simulink library "halin"  (R2021b)
settings: Solver=VariableStepAuto  StartTime=0.0  StopTime=10.0  RelTol=1e-3
undefined symbols (not defined in the file): KHAL_CAN1ABM1E2E_flg, KHAL_CAN1ESC1E2E_flg, KHAL_CAN1ESC5E2E_flg, KHAL_CAN1ESC7E2E_flg, KHAL_CAN1FCM2E2E_flg, KHAL_CAN1FCM3E2E_flg, KHAL_CAN1FCM4E2E_flg, KHAL_CAN3BMS1E2E_flg, KHAL_CAN3BMS6E2E_flg, KHAL_CAN3CCU1E2E_flg, KHAL_CAN3CCU2E2E_flg, KHAL_CAN3MCUF1E2E_flg, KHAL_CAN3MCUR1E2E_flg, KHAL_CAN3Shifter1E2E_flg, TRUE
libraries: simulink x420, FVT_lib x149, hcu_lib x49
(part 10 of 14)

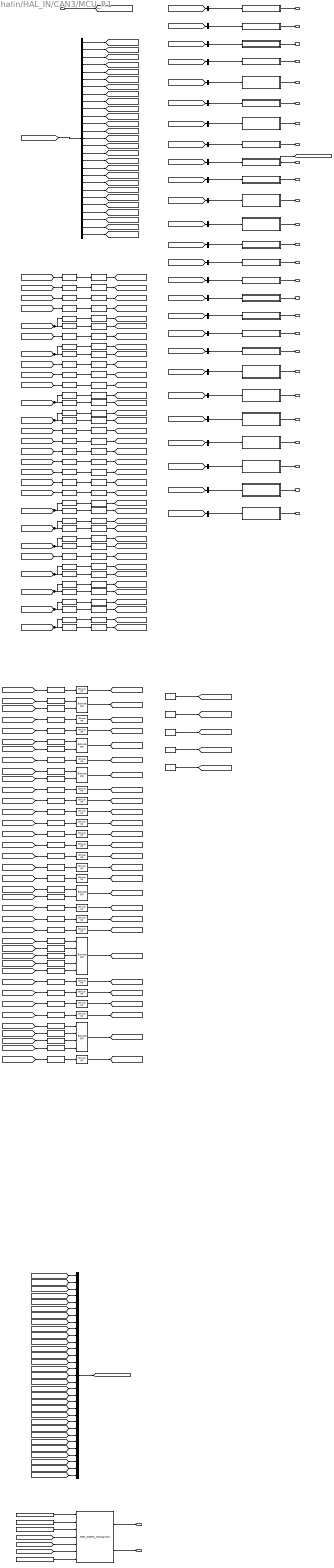
== system halin/HAL_IN/CAN3/MCU_R1 ==
  DT_CAN3_SG_MCU_R1 : Inport
  0x02 : Constant  Value=0x02
  0x78 : Constant  Value=0x78
  BitwiseAND{,1..37} (38 alike) : simulink/Logic and Bit Operations/Bitwise Operator  logicop=AND  UseBitMask=on  BitMask=0xFF  BitMaskRealWorld=Stored Integer
  BitwiseOR{,2..3,5,7..15,17..19,21..24,26} (21 alike) : simulink/Logic and Bit Operations/Bitwise Operator  logicop=OR  UseBitMask=off  BitMask=bin2dec('11011001')  BitMaskRealWorld=Stored Integer
  BitwiseOR{1,4,6,16} (4 alike) : simulink/Logic and Bit Operations/Bitwise Operator  logicop=OR  UseBitMask=off  NumInputPorts=2  BitMask=bin2dec('11011001')  BitMaskRealWorld=Stored Integer
  BitwiseOR20 : simulink/Logic and Bit Operations/Bitwise Operator  logicop=OR  UseBitMask=off  NumInputPorts=5  BitMask=bin2dec('11011001')  BitMaskRealWorld=Stored Integer
  BitwiseOR25 : simulink/Logic and Bit Operations/Bitwise Operator  logicop=OR  UseBitMask=off  NumInputPorts=4  BitMask=bin2dec('11011001')  BitMaskRealWorld=Stored Integer
  DDM_CS&RC_Comparison : FVT_lib/hal/DDM_CS&RC_Comparison  MsgCycleTime=10
  Data Type Conversion{,1..37} (38 alike) : DataTypeConversion  OutDataTypeStr=uint8
  KHAL_CAN3MCUR1E2E_flg : Constant  Value=KHAL_CAN3MCUR1E2E_flg
  LeftShift{,5,7,10..11,13..14} (7 alike) : ArithShift  BitShiftDirection=Left
  LeftShift1 : ArithShift  BitShiftNumber=1  BitShiftDirection=Left
  LeftShift12 : ArithShift  BitShiftNumber=7  BitShiftDirection=Left
  LeftShift15 : ArithShift  BitShiftNumber=1  BitShiftDirection=Left
  LeftShift2 : ArithShift  BitShiftNumber=2  BitShiftDirection=Left
  LeftShift3 : ArithShift  BitShiftNumber=5  BitShiftDirection=Left
  LeftShift4 : ArithShift  BitShiftNumber=6  BitShiftDirection=Left
  LeftShift6 : ArithShift  BitShiftNumber=4  BitShiftDirection=Left
  LeftShift8 : ArithShift  BitShiftNumber=3  BitShiftDirection=Left
  LeftShift9 : ArithShift  BitShiftNumber=4  BitShiftDirection=Left
  MCUWarnR : Subsystem
  MessageRollingCounter : FVT_lib/hal/MessageRollingCounter  CounterMAX=14  task_time_ms=5  msg_time_ms=10
  Mux : Mux  Inputs=31
  RightShift{,2,4,6,10,14,16,18,20} (9 alike) : ArithShift  BitShiftNumber=8
  RightShift{1,3,5,7,11,15,17,19,21} (9 alike) : ArithShift
  RightShift12 : ArithShift  BitShiftNumber=4
  RightShift13 : ArithShift  BitShiftNumber=-4
  RightShift8 : ArithShift  BitShiftNumber=1
  RightShift9 : ArithShift  BitShiftNumber=-7
  RrActvDmpDisabSta : Subsystem
  RrEDUDrtSta : Subsystem
  RrEDUOpratingSta : Subsystem
  RrEDURealTMTq : Subsystem
  RrEDURotateDirction : Subsystem
  RrEDUTqReqFbk : Subsystem
  RrMCU1Chksum : Subsystem
  RrMCU1RolCnt : Subsystem
  RrMCUBAT : Subsystem
  RrMCUDCBusCurr : Subsystem
  RrMCUDCBusVolt : Subsystem
  RrMCUDischrgSta : Subsystem
  RrMCUEnaSta : Subsystem
  RrMCUErr : Subsystem
  RrMCUIGNsta : Subsystem
  RrMCUReady : Subsystem
  RrMCUReady4Pre : Subsystem
  RrMCUSysSta : Subsystem
  RrMCUTemp : Subsystem
  RrMotorAvailTq : Subsystem
  RrRegenAvailTq : Subsystem
  RrTMSpd : Subsystem
  RrTMTemp : Subsystem
  RrTMid : Subsystem
  RrTMiq : Subsystem
  bus_selector : BusSelector  OutputSignals=CAN3_MCUWarn_R,CAN3_Rr_ActvDmpDisabSta,CAN3_Rr_EDUDrtSta,CAN3_Rr_EDUOpratingSta,CAN3_Rr_EDURealTMTq,CAN3_Rr_EDURotateDirction,CAN3_Rr_EDUTqReqFbk,CAN3_Rr_MCU1Chksum,CAN3_Rr_MCU1RolCnt,CAN3_Rr_MCUBAT,CAN3_Rr_MCUDCBusCurr,CAN3_Rr_MCUDCBusVolt,CAN3_Rr_MCUDischrgSta,CAN3_Rr_MCUEnaSta,CAN3_Rr_MCUErr,CAN3_Rr_MCUIGN_sta,CAN3_Rr_MCUReady,CAN3_Rr_MCUReady4Pre,CAN3_Rr_MCUSysSta,CAN3_Rr_MCUTemp,CAN3_Rr_MotorAvailTq,CAN3_Rr_RegenAvailTq,CAN3_Rr_Reserved_bits,CAN3_Rr_TMSpd,CAN3_Rr_TMTemp,CAN3_Rr_TMid,CAN3_Rr_TMiq
  bus_selector1 : BusSelector  OutputSignals=CAN3_MCUWarn_R
  bus_selector10 : BusSelector  OutputSignals=CAN3_Rr_MCUBAT
  bus_selector11 : BusSelector  OutputSignals=CAN3_Rr_MCUDCBusCurr
  bus_selector12 : BusSelector  OutputSignals=CAN3_Rr_MCUDCBusVolt
  bus_selector13 : BusSelector  OutputSignals=CAN3_Rr_MCUDischrgSta
  bus_selector14 : BusSelector  OutputSignals=CAN3_Rr_MCUEnaSta
  bus_selector15 : BusSelector  OutputSignals=CAN3_Rr_MCUErr
  bus_selector16 : BusSelector  OutputSignals=CAN3_Rr_MCUIGN_sta
  bus_selector17 : BusSelector  OutputSignals=CAN3_Rr_MCUReady
  bus_selector18 : BusSelector  OutputSignals=CAN3_Rr_MCUReady4Pre
  bus_selector19 : BusSelector  OutputSignals=CAN3_Rr_MCUSysSta
  bus_selector2 : BusSelector  OutputSignals=CAN3_Rr_ActvDmpDisabSta
  bus_selector20 : BusSelector  OutputSignals=CAN3_Rr_MCUTemp
  bus_selector21 : BusSelector  OutputSignals=CAN3_Rr_MotorAvailTq
  bus_selector22 : BusSelector  OutputSignals=CAN3_Rr_RegenAvailTq
  bus_selector23 : BusSelector  OutputSignals=CAN3_Rr_TMSpd
  bus_selector24 : BusSelector  OutputSignals=CAN3_Rr_TMTemp
  bus_selector25 : BusSelector  OutputSignals=CAN3_Rr_TMid
  bus_selector26 : BusSelector  OutputSignals=CAN3_Rr_TMiq
  bus_selector3 : BusSelector  OutputSignals=CAN3_Rr_EDUDrtSta
  bus_selector4 : BusSelector  OutputSignals=CAN3_Rr_EDUOpratingSta
  bus_selector5 : BusSelector  OutputSignals=CAN3_Rr_EDURealTMTq
  bus_selector6 : BusSelector  OutputSignals=CAN3_Rr_EDURotateDirction
  bus_selector7 : BusSelector  OutputSignals=CAN3_Rr_EDUTqReqFbk
  bus_selector8 : BusSelector  OutputSignals=CAN3_Rr_MCU1Chksum
  bus_selector9 : BusSelector  OutputSignals=CAN3_Rr_MCU1RolCnt
  constant{,1..4} (5 alike) : Constant  Value=0x0  OutDataTypeStr=uint8
  VHAL_MCUR1CSErr_flg : Outport
  VHAL_MCUR1RCErr_flg : Outport  Port=2
  VHAL_MCUWarnR_enum : Outport  Port=3
  VHAL_RrActvDmpDisabSta_flg : Outport  Port=4
  VHAL_RrEDUDrtSta_flg : Outport  Port=5
  VHAL_RrEDUOpratingSta_flg : Outport  Port=6
  VHAL_RrEDURealTMTq_Nm : Outport  Port=7
  VHAL_RrEDURotateDirction_enum : Outport  Port=8
  VHAL_RrEDUTqReqFbk_Nm : Outport  Port=9
  VHAL_RrMCU1Chksum_enum : Outport  Port=10
  VHAL_RrMCU1RolCnt_enum : Outport  Port=11
  VHAL_RrMCUBAT_V : Outport  Port=12
  VHAL_RrMCUDCBusCurr_A : Outport  Port=13
  VHAL_RrMCUDCBusVolt_V : Outport  Port=14
  VHAL_RrMCUDischrgSta_flg : Outport  Port=15
  VHAL_RrMCUEnaSta_flg : Outport  Port=16
  VHAL_RrMCUErr_enum : Outport  Port=17
  VHAL_RrMCUIGNsta_flg : Outport  Port=18
  VHAL_RrMCUReady_flg : Outport  Port=19
  VHAL_RrMCUReady4Pre_flg : Outport  Port=20
  VHAL_RrMCUSysSta_enum : Outport  Port=21
  VHAL_RrMCUTemp_C : Outport  Port=22
  VHAL_RrMotorAvailTq_Nm : Outport  Port=23
  VHAL_RrRegenAvailTq_Nm : Outport  Port=24
  VHAL_RrTMSpd_rpm : Outport  Port=25
  VHAL_RrTMTemp_C : Outport  Port=26
  VHAL_RrTMid_A : Outport  Port=27
  VHAL_RrTMiq_A : Outport  Port=28
  wires:
  DT_CAN3_SG_MCU_R1/1 -> [DT_CAN3_SG_MCU_R1]
  [DT_CAN3_SG_MCU_R1] -> bus_selector/1
  bus_selector/1 -> [CAN3_MCUWarn_R]  "<CAN3_MCUWarn_R>"
  [CAN3_MCUWarn_R] -> LeftShift/1
  LeftShift/1 -> BitwiseAND/1
  BitwiseAND/1 -> [Byte_1_CAN3_MCUWarn_R]
  bus_selector/2 -> [CAN3_Rr_ActvDmpDisabSta]  "<CAN3_Rr_ActvDmpDisabSta>"
  [CAN3_Rr_ActvDmpDisabSta] -> LeftShift1/1
  LeftShift1/1 -> BitwiseAND1/1
  BitwiseAND1/1 -> [Byte_25_CAN3_Rr_ActvDmpDisabSta]
  bus_selector/3 -> [CAN3_Rr_EDUDrtSta]  "<CAN3_Rr_EDUDrtSta>"
  [CAN3_Rr_EDUDrtSta] -> LeftShift2/1
  LeftShift2/1 -> BitwiseAND2/1
  BitwiseAND2/1 -> [Byte_25_CAN3_Rr_EDUDrtSta]
  bus_selector/4 -> [CAN3_Rr_EDUOpratingSta]  "<CAN3_Rr_EDUOpratingSta>"
  [CAN3_Rr_EDUOpratingSta] -> LeftShift3/1
  LeftShift3/1 -> BitwiseAND3/1
  BitwiseAND3/1 -> [Byte_30_CAN3_Rr_EDUOpratingSta]
  bus_selector/5 -> [CAN3_Rr_EDURealTMTq]  "<CAN3_Rr_EDURealTMTq>"
  [CAN3_Rr_EDURealTMTq] -> RightShift/1, RightShift1/1
  RightShift/1 -> BitwiseAND4/1
  BitwiseAND4/1 -> [Byte_28_CAN3_Rr_EDURealTMTq]
  RightShift1/1 -> BitwiseAND5/1
  BitwiseAND5/1 -> [Byte_29_CAN3_Rr_EDURealTMTq]
  bus_selector/6 -> [CAN3_Rr_EDURotateDirction]  "<CAN3_Rr_EDURotateDirction>"
  [CAN3_Rr_EDURotateDirction] -> LeftShift4/1
  LeftShift4/1 -> BitwiseAND6/1
  BitwiseAND6/1 -> [Byte_30_CAN3_Rr_EDURotateDirction]
  bus_selector/7 -> [CAN3_Rr_EDUTqReqFbk]  "<CAN3_Rr_EDUTqReqFbk>"
  [CAN3_Rr_EDUTqReqFbk] -> RightShift2/1, RightShift3/1
  RightShift2/1 -> BitwiseAND7/1
  BitwiseAND7/1 -> [Byte_30_CAN3_Rr_EDUTqReqFbk]
  RightShift3/1 -> BitwiseAND8/1
  BitwiseAND8/1 -> [Byte_31_CAN3_Rr_EDUTqReqFbk]
  bus_selector/8 -> [CAN3_Rr_MCU1Chksum]  "<CAN3_Rr_MCU1Chksum>"
  [CAN3_Rr_MCU1Chksum] -> LeftShift5/1
  LeftShift5/1 -> BitwiseAND9/1
  BitwiseAND9/1 -> [Byte_0_CAN3_Rr_MCU1Chksum]
  bus_selector/9 -> [CAN3_Rr_MCU1RolCnt]  "<CAN3_Rr_MCU1RolCnt>"
  [CAN3_Rr_MCU1RolCnt] -> LeftShift6/1
  LeftShift6/1 -> BitwiseAND10/1
  BitwiseAND10/1 -> [Byte_1_CAN3_Rr_MCU1RolCnt]
  bus_selector/10 -> [CAN3_Rr_MCUBAT]  "<CAN3_Rr_MCUBAT>"
  [CAN3_Rr_MCUBAT] -> LeftShift7/1
  LeftShift7/1 -> BitwiseAND11/1
  BitwiseAND11/1 -> [Byte_8_CAN3_Rr_MCUBAT]
  bus_selector/11 -> [CAN3_Rr_MCUDCBusCurr]  "<CAN3_Rr_MCUDCBusCurr>"
  [CAN3_Rr_MCUDCBusCurr] -> RightShift4/1, RightShift5/1
  RightShift4/1 -> BitwiseAND12/1
  BitwiseAND12/1 -> [Byte_21_CAN3_Rr_MCUDCBusCurr]
  RightShift5/1 -> BitwiseAND13/1
  BitwiseAND13/1 -> [Byte_22_CAN3_Rr_MCUDCBusCurr]
  bus_selector/12 -> [CAN3_Rr_MCUDCBusVolt]  "<CAN3_Rr_MCUDCBusVolt>"
  [CAN3_Rr_MCUDCBusVolt] -> RightShift6/1, RightShift7/1
  RightShift6/1 -> BitwiseAND14/1
  BitwiseAND14/1 -> [Byte_23_CAN3_Rr_MCUDCBusVolt]
  RightShift7/1 -> BitwiseAND15/1
  BitwiseAND15/1 -> [Byte_24_CAN3_Rr_MCUDCBusVolt]
  bus_selector/13 -> [CAN3_Rr_MCUDischrgSta]  "<CAN3_Rr_MCUDischrgSta>"
  [CAN3_Rr_MCUDischrgSta] -> LeftShift8/1
  LeftShift8/1 -> BitwiseAND16/1
  BitwiseAND16/1 -> [Byte_25_CAN3_Rr_MCUDischrgSta]
  bus_selector/14 -> [CAN3_Rr_MCUEnaSta]  "<CAN3_Rr_MCUEnaSta>"
  [CAN3_Rr_MCUEnaSta] -> LeftShift9/1
  LeftShift9/1 -> BitwiseAND17/1
  BitwiseAND17/1 -> [Byte_30_CAN3_Rr_MCUEnaSta]
  bus_selector/15 -> [CAN3_Rr_MCUErr]  "<CAN3_Rr_MCUErr>"
  [CAN3_Rr_MCUErr] -> LeftShift10/1
  LeftShift10/1 -> BitwiseAND18/1
  BitwiseAND18/1 -> [Byte_17_CAN3_Rr_MCUErr]
  bus_selector/16 -> [CAN3_Rr_MCUIGN_sta]  "<CAN3_Rr_MCUIGN_sta>"
  [CAN3_Rr_MCUIGN_sta] -> LeftShift11/1
  LeftShift11/1 -> BitwiseAND19/1
  BitwiseAND19/1 -> [Byte_9_CAN3_Rr_MCUIGN_sta]
  bus_selector/17 -> [CAN3_Rr_MCUReady]  "<CAN3_Rr_MCUReady>"
  [CAN3_Rr_MCUReady] -> LeftShift12/1
  LeftShift12/1 -> BitwiseAND20/1
  BitwiseAND20/1 -> [Byte_25_CAN3_Rr_MCUReady]
  bus_selector/18 -> [CAN3_Rr_MCUReady4Pre]  "<CAN3_Rr_MCUReady4Pre>"
  [CAN3_Rr_MCUReady4Pre] -> LeftShift13/1
  LeftShift13/1 -> BitwiseAND21/1
  BitwiseAND21/1 -> [Byte_25_CAN3_Rr_MCUReady4Pre]
  bus_selector/19 -> [CAN3_Rr_MCUSysSta]  "<CAN3_Rr_MCUSysSta>"
  [CAN3_Rr_MCUSysSta] -> LeftShift14/1
  LeftShift14/1 -> BitwiseAND22/1
  BitwiseAND22/1 -> [Byte_7_CAN3_Rr_MCUSysSta]
  bus_selector/20 -> [CAN3_Rr_MCUTemp]  "<CAN3_Rr_MCUTemp>"
  [CAN3_Rr_MCUTemp] -> RightShift8/1, RightShift9/1
  RightShift8/1 -> BitwiseAND23/1
  BitwiseAND23/1 -> [Byte_20_CAN3_Rr_MCUTemp]
  RightShift9/1 -> BitwiseAND24/1
  BitwiseAND24/1 -> [Byte_21_CAN3_Rr_MCUTemp]
  bus_selector/21 -> [CAN3_Rr_MotorAvailTq]  "<CAN3_Rr_MotorAvailTq>"
  [CAN3_Rr_MotorAvailTq] -> RightShift10/1, RightShift11/1
  RightShift10/1 -> BitwiseAND25/1
  BitwiseAND25/1 -> [Byte_11_CAN3_Rr_MotorAvailTq]
  RightShift11/1 -> BitwiseAND26/1
  BitwiseAND26/1 -> [Byte_12_CAN3_Rr_MotorAvailTq]
  bus_selector/22 -> [CAN3_Rr_RegenAvailTq]  "<CAN3_Rr_RegenAvailTq>"
  [CAN3_Rr_RegenAvailTq] -> RightShift12/1, RightShift13/1
  RightShift12/1 -> BitwiseAND27/1
  BitwiseAND27/1 -> [Byte_10_CAN3_Rr_RegenAvailTq]
  RightShift13/1 -> BitwiseAND28/1
  BitwiseAND28/1 -> [Byte_11_CAN3_Rr_RegenAvailTq]
  bus_selector/23 -> [CAN3_Rr_Reserved_bits]  "<CAN3_Rr_Reserved_bits>"
  [CAN3_Rr_Reserved_bits] -> LeftShift15/1
  LeftShift15/1 -> BitwiseAND29/1
  BitwiseAND29/1 -> [Byte_9_CAN3_Rr_Reserved_bits]
  bus_selector/24 -> [CAN3_Rr_TMSpd]  "<CAN3_Rr_TMSpd>"
  [CAN3_Rr_TMSpd] -> RightShift14/1, RightShift15/1
  RightShift14/1 -> BitwiseAND30/1
  BitwiseAND30/1 -> [Byte_26_CAN3_Rr_TMSpd]
  RightShift15/1 -> BitwiseAND31/1
  BitwiseAND31/1 -> [Byte_27_CAN3_Rr_TMSpd]
  bus_selector/25 -> [CAN3_Rr_TMTemp]  "<CAN3_Rr_TMTemp>"
  [CAN3_Rr_TMTemp] -> RightShift16/1, RightShift17/1
  RightShift16/1 -> BitwiseAND32/1
  BitwiseAND32/1 -> [Byte_18_CAN3_Rr_TMTemp]
  RightShift17/1 -> BitwiseAND33/1
  BitwiseAND33/1 -> [Byte_19_CAN3_Rr_TMTemp]
  bus_selector/26 -> [CAN3_Rr_TMid]  "<CAN3_Rr_TMid>"
  [CAN3_Rr_TMid] -> RightShift18/1, RightShift19/1
  RightShift18/1 -> BitwiseAND34/1
  BitwiseAND34/1 -> [Byte_15_CAN3_Rr_TMid]
  RightShift19/1 -> BitwiseAND35/1
  BitwiseAND35/1 -> [Byte_16_CAN3_Rr_TMid]
  bus_selector/27 -> [CAN3_Rr_TMiq]  "<CAN3_Rr_TMiq>"
  [CAN3_Rr_TMiq] -> RightShift20/1, RightShift21/1
  RightShift20/1 -> BitwiseAND36/1
  BitwiseAND36/1 -> [Byte_13_CAN3_Rr_TMiq]
  RightShift21/1 -> BitwiseAND37/1
  BitwiseAND37/1 -> [Byte_14_CAN3_Rr_TMiq]
  Data Type Conversion/1 -> BitwiseOR/1
  [Byte_0_CAN3_Rr_MCU1Chksum] -> Data Type Conversion/1
  BitwiseOR/1 -> [Byte_0]
  Data Type Conversion1/1 -> BitwiseOR1/1
  [Byte_1_CAN3_MCUWarn_R] -> Data Type Conversion1/1
  Data Type Conversion2/1 -> BitwiseOR1/2
  [Byte_1_CAN3_Rr_MCU1RolCnt] -> Data Type Conversion2/1
  BitwiseOR1/1 -> [Byte_1]
  constant/1 -> [Byte_2]
  constant1/1 -> [Byte_3]
  constant2/1 -> [Byte_4]
  constant3/1 -> [Byte_5]
  constant4/1 -> [Byte_6]
  Data Type Conversion3/1 -> BitwiseOR2/1
  [Byte_7_CAN3_Rr_MCUSysSta] -> Data Type Conversion3/1
  BitwiseOR2/1 -> [Byte_7]
  Data Type Conversion4/1 -> BitwiseOR3/1
  [Byte_8_CAN3_Rr_MCUBAT] -> Data Type Conversion4/1
  BitwiseOR3/1 -> [Byte_8]
  Data Type Conversion5/1 -> BitwiseOR4/1
  [Byte_9_CAN3_Rr_MCUIGN_sta] -> Data Type Conversion5/1
  Data Type Conversion6/1 -> BitwiseOR4/2
  [Byte_9_CAN3_Rr_Reserved_bits] -> Data Type Conversion6/1
  BitwiseOR4/1 -> [Byte_9]
  Data Type Conversion7/1 -> BitwiseOR5/1
  [Byte_10_CAN3_Rr_RegenAvailTq] -> Data Type Conversion7/1
  BitwiseOR5/1 -> [Byte_10]
  Data Type Conversion8/1 -> BitwiseOR6/1
  [Byte_11_CAN3_Rr_MotorAvailTq] -> Data Type Conversion8/1
  Data Type Conversion9/1 -> BitwiseOR6/2
  [Byte_11_CAN3_Rr_RegenAvailTq] -> Data Type Conversion9/1
  BitwiseOR6/1 -> [Byte_11]
  Data Type Conversion10/1 -> BitwiseOR7/1
  [Byte_12_CAN3_Rr_MotorAvailTq] -> Data Type Conversion10/1
  BitwiseOR7/1 -> [Byte_12]
  Data Type Conversion11/1 -> BitwiseOR8/1
  [Byte_13_CAN3_Rr_TMiq] -> Data Type Conversion11/1
  BitwiseOR8/1 -> [Byte_13]
  Data Type Conversion12/1 -> BitwiseOR9/1
  [Byte_14_CAN3_Rr_TMiq] -> Data Type Conversion12/1
  BitwiseOR9/1 -> [Byte_14]
  Data Type Conversion13/1 -> BitwiseOR10/1
  [Byte_15_CAN3_Rr_TMid] -> Data Type Conversion13/1
  BitwiseOR10/1 -> [Byte_15]
  Data Type Conversion14/1 -> BitwiseOR11/1
  [Byte_16_CAN3_Rr_TMid] -> Data Type Conversion14/1
  BitwiseOR11/1 -> [Byte_16]
  Data Type Conversion15/1 -> BitwiseOR12/1
  [Byte_17_CAN3_Rr_MCUErr] -> Data Type Conversion15/1
  BitwiseOR12/1 -> [Byte_17]
  Data Type Conversion16/1 -> BitwiseOR13/1
  [Byte_18_CAN3_Rr_TMTemp] -> Data Type Conversion16/1
  BitwiseOR13/1 -> [Byte_18]
  Data Type Conversion17/1 -> BitwiseOR14/1
  [Byte_19_CAN3_Rr_TMTemp] -> Data Type Conversion17/1
  BitwiseOR14/1 -> [Byte_19]
  Data Type Conversion18/1 -> BitwiseOR15/1
  [Byte_20_CAN3_Rr_MCUTemp] -> Data Type Conversion18/1
  BitwiseOR15/1 -> [Byte_20]
  Data Type Conversion19/1 -> BitwiseOR16/1
  [Byte_21_CAN3_Rr_MCUDCBusCurr] -> Data Type Conversion19/1
  Data Type Conversion20/1 -> BitwiseOR16/2
  [Byte_21_CAN3_Rr_MCUTemp] -> Data Type Conversion20/1
  BitwiseOR16/1 -> [Byte_21]
  Data Type Conversion21/1 -> BitwiseOR17/1
  [Byte_22_CAN3_Rr_MCUDCBusCurr] -> Data Type Conversion21/1
  BitwiseOR17/1 -> [Byte_22]
  Data Type Conversion22/1 -> BitwiseOR18/1
  [Byte_23_CAN3_Rr_MCUDCBusVolt] -> Data Type Conversion22/1
  BitwiseOR18/1 -> [Byte_23]
  Data Type Conversion23/1 -> BitwiseOR19/1
  [Byte_24_CAN3_Rr_MCUDCBusVolt] -> Data Type Conversion23/1
  BitwiseOR19/1 -> [Byte_24]
  Data Type Conversion24/1 -> BitwiseOR20/1
  [Byte_25_CAN3_Rr_ActvDmpDisabSta] -> Data Type Conversion24/1
  Data Type Conversion25/1 -> BitwiseOR20/2
  [Byte_25_CAN3_Rr_EDUDrtSta] -> Data Type Conversion25/1
  Data Type Conversion26/1 -> BitwiseOR20/3
  [Byte_25_CAN3_Rr_MCUDischrgSta] -> Data Type Conversion26/1
  Data Type Conversion27/1 -> BitwiseOR20/4
  [Byte_25_CAN3_Rr_MCUReady] -> Data Type Conversion27/1
  Data Type Conversion28/1 -> BitwiseOR20/5
  [Byte_25_CAN3_Rr_MCUReady4Pre] -> Data Type Conversion28/1
  BitwiseOR20/1 -> [Byte_25]
  Data Type Conversion29/1 -> BitwiseOR21/1
  [Byte_26_CAN3_Rr_TMSpd] -> Data Type Conversion29/1
  BitwiseOR21/1 -> [Byte_26]
  Data Type Conversion30/1 -> BitwiseOR22/1
  [Byte_27_CAN3_Rr_TMSpd] -> Data Type Conversion30/1
  BitwiseOR22/1 -> [Byte_27]
  Data Type Conversion31/1 -> BitwiseOR23/1
  [Byte_28_CAN3_Rr_EDURealTMTq] -> Data Type Conversion31/1
  BitwiseOR23/1 -> [Byte_28]
  Data Type Conversion32/1 -> BitwiseOR24/1
  [Byte_29_CAN3_Rr_EDURealTMTq] -> Data Type Conversion32/1
  BitwiseOR24/1 -> [Byte_29]
  Data Type Conversion33/1 -> BitwiseOR25/1
  [Byte_30_CAN3_Rr_EDUOpratingSta] -> Data Type Conversion33/1
  Data Type Conversion34/1 -> BitwiseOR25/2
  [Byte_30_CAN3_Rr_EDURotateDirction] -> Data Type Conversion34/1
  Data Type Conversion35/1 -> BitwiseOR25/3
  [Byte_30_CAN3_Rr_EDUTqReqFbk] -> Data Type Conversion35/1
  Data Type Conversion36/1 -> BitwiseOR25/4
  [Byte_30_CAN3_Rr_MCUEnaSta] -> Data Type Conversion36/1
  BitwiseOR25/1 -> [Byte_30]
  Data Type Conversion37/1 -> BitwiseOR26/1
  [Byte_31_CAN3_Rr_EDUTqReqFbk] -> Data Type Conversion37/1
  BitwiseOR26/1 -> [Byte_31]
  [Byte_1] -> Mux/1
  [Byte_2] -> Mux/2
  [Byte_3] -> Mux/3
  [Byte_4] -> Mux/4
  [Byte_5] -> Mux/5
  [Byte_6] -> Mux/6
  [Byte_7] -> Mux/7
  [Byte_8] -> Mux/8
  [Byte_9] -> Mux/9
  [Byte_10] -> Mux/10
  [Byte_11] -> Mux/11
  [Byte_12] -> Mux/12
  [Byte_13] -> Mux/13
  [Byte_14] -> Mux/14
  [Byte_15] -> Mux/15
  [Byte_16] -> Mux/16
  [Byte_17] -> Mux/17
  [Byte_18] -> Mux/18
  [Byte_19] -> Mux/19
  [Byte_20] -> Mux/20
  [Byte_21] -> Mux/21
  [Byte_22] -> Mux/22
  [Byte_23] -> Mux/23
  [Byte_24] -> Mux/24
  [Byte_25] -> Mux/25
  [Byte_26] -> Mux/26
  [Byte_27] -> Mux/27
  [Byte_28] -> Mux/28
  [Byte_29] -> Mux/29
  [Byte_30] -> Mux/30
  [Byte_31] -> Mux/31
  Mux/1 -> [VHAL_CAN3MCUR1noCS_raw]
  KHAL_CAN3MCUR1E2E_flg/1 -> DDM_CS&RC_Comparison/1
  0x78/1 -> DDM_CS&RC_Comparison/2
  0x02/1 -> DDM_CS&RC_Comparison/3
  [VHAL_CAN3MCUR1noCS_raw] -> DDM_CS&RC_Comparison/4
  [Byte_0] -> DDM_CS&RC_Comparison/5
  [RC_ECU] -> DDM_CS&RC_Comparison/6
  MessageRollingCounter/1 -> DDM_CS&RC_Comparison/7
  DDM_CS&RC_Comparison/1 -> VHAL_MCUR1CSErr_flg/1
  DDM_CS&RC_Comparison/2 -> VHAL_MCUR1RCErr_flg/1
  [DT_CAN3_SG_MCU_R1] -> bus_selector1/1
  bus_selector1/1 -> MCUWarnR/1(MCUWarn_R)  "<CAN3_MCUWarn_R>"
  MCUWarnR/1(VHAL_MCUWarnR_enum) -> VHAL_MCUWarnR_enum/1
  [DT_CAN3_SG_MCU_R1] -> bus_selector2/1
  bus_selector2/1 -> RrActvDmpDisabSta/1(Rr_ActvDmpDisabSta)  "<CAN3_Rr_ActvDmpDisabSta>"
  RrActvDmpDisabSta/1(VHAL_RrActvDmpDisabSta_flg) -> VHAL_RrActvDmpDisabSta_flg/1
  [DT_CAN3_SG_MCU_R1] -> bus_selector3/1
  bus_selector3/1 -> RrEDUDrtSta/1(Rr_EDUDrtSta)  "<CAN3_Rr_EDUDrtSta>"
  RrEDUDrtSta/1(VHAL_RrEDUDrtSta_flg) -> VHAL_RrEDUDrtSta_flg/1
  [DT_CAN3_SG_MCU_R1] -> bus_selector4/1
  bus_selector4/1 -> RrEDUOpratingSta/1(Rr_EDUOpratingSta)  "<CAN3_Rr_EDUOpratingSta>"
  RrEDUOpratingSta/1(VHAL_RrEDUOpratingSta_flg) -> VHAL_RrEDUOpratingSta_flg/1
  [DT_CAN3_SG_MCU_R1] -> bus_selector5/1
  bus_selector5/1 -> RrEDURealTMTq/1(Rr_EDURealTMTq)  "<CAN3_Rr_EDURealTMTq>"
  RrEDURealTMTq/1(VHAL_RrEDURealTMTq_Nm) -> VHAL_RrEDURealTMTq_Nm/1
  [DT_CAN3_SG_MCU_R1] -> bus_selector6/1
  bus_selector6/1 -> RrEDURotateDirction/1(Rr_EDURotateDirction)  "<CAN3_Rr_EDURotateDirction>"
  RrEDURotateDirction/1(VHAL_RrEDURotateDirction_enum) -> VHAL_RrEDURotateDirction_enum/1
  [DT_CAN3_SG_MCU_R1] -> bus_selector7/1
  bus_selector7/1 -> RrEDUTqReqFbk/1(Rr_EDUTqReqFbk)  "<CAN3_Rr_EDUTqReqFbk>"
  RrEDUTqReqFbk/1(VHAL_RrEDUTqReqFbk_Nm) -> VHAL_RrEDUTqReqFbk_Nm/1
  [DT_CAN3_SG_MCU_R1] -> bus_selector8/1
  bus_selector8/1 -> RrMCU1Chksum/1(Rr_MCU1Chksum)  "<CAN3_Rr_MCU1Chksum>"
  RrMCU1Chksum/1(VHAL_RrMCU1Chksum_enum) -> VHAL_RrMCU1Chksum_enum/1
  [DT_CAN3_SG_MCU_R1] -> bus_selector9/1
  bus_selector9/1 -> RrMCU1RolCnt/1(Rr_MCU1RolCnt)  "<CAN3_Rr_MCU1RolCnt>"
  RrMCU1RolCnt/1(VHAL_RrMCU1RolCnt_enum) -> VHAL_RrMCU1RolCnt_enum/1, [RC_ECU]
  [DT_CAN3_SG_MCU_R1] -> bus_selector10/1
  bus_selector10/1 -> RrMCUBAT/1(Rr_MCUBAT)  "<CAN3_Rr_MCUBAT>"
  RrMCUBAT/1(VHAL_RrMCUBAT_V) -> VHAL_RrMCUBAT_V/1
  [DT_CAN3_SG_MCU_R1] -> bus_selector11/1
  bus_selector11/1 -> RrMCUDCBusCurr/1(Rr_MCUDCBusCurr)  "<CAN3_Rr_MCUDCBusCurr>"
  RrMCUDCBusCurr/1(VHAL_RrMCUDCBusCurr_A) -> VHAL_RrMCUDCBusCurr_A/1
  [DT_CAN3_SG_MCU_R1] -> bus_selector12/1
  bus_selector12/1 -> RrMCUDCBusVolt/1(Rr_MCUDCBusVolt)  "<CAN3_Rr_MCUDCBusVolt>"
  RrMCUDCBusVolt/1(VHAL_RrMCUDCBusVolt_V) -> VHAL_RrMCUDCBusVolt_V/1
  [DT_CAN3_SG_MCU_R1] -> bus_selector13/1
  bus_selector13/1 -> RrMCUDischrgSta/1(Rr_MCUDischrgSta)  "<CAN3_Rr_MCUDischrgSta>"
  RrMCUDischrgSta/1(VHAL_RrMCUDischrgSta_flg) -> VHAL_RrMCUDischrgSta_flg/1
  [DT_CAN3_SG_MCU_R1] -> bus_selector14/1
  bus_selector14/1 -> RrMCUEnaSta/1(Rr_MCUEnaSta)  "<CAN3_Rr_MCUEnaSta>"
  RrMCUEnaSta/1(VHAL_RrMCUEnaSta_flg) -> VHAL_RrMCUEnaSta_flg/1
  [DT_CAN3_SG_MCU_R1] -> bus_selector15/1
  bus_selector15/1 -> RrMCUErr/1(Rr_MCUErr)  "<CAN3_Rr_MCUErr>"
  RrMCUErr/1(VHAL_RrMCUErr_enum) -> VHAL_RrMCUErr_enum/1
  [DT_CAN3_SG_MCU_R1] -> bus_selector16/1
  bus_selector16/1 -> RrMCUIGNsta/1(Rr_MCUIGN_sta)  "<CAN3_Rr_MCUIGN_sta>"
  RrMCUIGNsta/1(VHAL_RrMCUIGNsta_flg) -> VHAL_RrMCUIGNsta_flg/1
  [DT_CAN3_SG_MCU_R1] -> bus_selector17/1
  bus_selector17/1 -> RrMCUReady/1(Rr_MCUReady)  "<CAN3_Rr_MCUReady>"
  RrMCUReady/1(VHAL_RrMCUReady_flg) -> VHAL_RrMCUReady_flg/1
  [DT_CAN3_SG_MCU_R1] -> bus_selector18/1
  bus_selector18/1 -> RrMCUReady4Pre/1(Rr_MCUReady4Pre)  "<CAN3_Rr_MCUReady4Pre>"
  RrMCUReady4Pre/1(VHAL_RrMCUReady4Pre_flg) -> VHAL_RrMCUReady4Pre_flg/1
  [DT_CAN3_SG_MCU_R1] -> bus_selector19/1
  bus_selector19/1 -> RrMCUSysSta/1(Rr_MCUSysSta)  "<CAN3_Rr_MCUSysSta>"
  RrMCUSysSta/1(VHAL_RrMCUSysSta_enum) -> VHAL_RrMCUSysSta_enum/1
  [DT_CAN3_SG_MCU_R1] -> bus_selector20/1
  bus_selector20/1 -> RrMCUTemp/1(Rr_MCUTemp)  "<CAN3_Rr_MCUTemp>"
  RrMCUTemp/1(VHAL_RrMCUTemp_C) -> VHAL_RrMCUTemp_C/1
  [DT_CAN3_SG_MCU_R1] -> bus_selector21/1
  bus_selector21/1 -> RrMotorAvailTq/1(Rr_MotorAvailTq)  "<CAN3_Rr_MotorAvailTq>"
  RrMotorAvailTq/1(VHAL_RrMotorAvailTq_Nm) -> VHAL_RrMotorAvailTq_Nm/1
  [DT_CAN3_SG_MCU_R1] -> bus_selector22/1
  bus_selector22/1 -> RrRegenAvailTq/1(Rr_RegenAvailTq)  "<CAN3_Rr_RegenAvailTq>"
  RrRegenAvailTq/1(VHAL_RrRegenAvailTq_Nm) -> VHAL_RrRegenAvailTq_Nm/1
  [DT_CAN3_SG_MCU_R1] -> bus_selector23/1
  bus_selector23/1 -> RrTMSpd/1(Rr_TMSpd)  "<CAN3_Rr_TMSpd>"
  RrTMSpd/1(VHAL_RrTMSpd_rpm) -> VHAL_RrTMSpd_rpm/1
  [DT_CAN3_SG_MCU_R1] -> bus_selector24/1
  bus_selector24/1 -> RrTMTemp/1(Rr_TMTemp)  "<CAN3_Rr_TMTemp>"
  RrTMTemp/1(VHAL_RrTMTemp_C) -> VHAL_RrTMTemp_C/1
  [DT_CAN3_SG_MCU_R1] -> bus_selector25/1
  bus_selector25/1 -> RrTMid/1(Rr_TMid)  "<CAN3_Rr_TMid>"
  RrTMid/1(VHAL_RrTMid_A) -> VHAL_RrTMid_A/1
  [DT_CAN3_SG_MCU_R1] -> bus_selector26/1
  bus_selector26/1 -> RrTMiq/1(Rr_TMiq)  "<CAN3_Rr_TMiq>"
  RrTMiq/1(VHAL_RrTMiq_A) -> VHAL_RrTMiq_A/1

== system halin/HAL_IN/CAN3/MCU_R2 ==
  DT_CAN3_SG_MCU_R2 : Inport
  RrCoolanttempReq : Subsystem
  RrEOPSpdSet : Subsystem
  RrFailcode1 : Subsystem
  RrFailcode2 : Subsystem
  RrFailcodehistory1 : Subsystem
  RrFailcodehistory2 : Subsystem
  RrLLCTemp : Subsystem
  RrLLCflowReq : Subsystem
  RrMCUTempWarn : Subsystem
  RrTMTempWarn : Subsystem
  bus_selector : BusSelector  OutputSignals=CAN3_Rr_CoolanttempReq
  bus_selector1 : BusSelector  OutputSignals=CAN3_Rr_EOP_SpdSet
  bus_selector2 : BusSelector  OutputSignals=CAN3_Rr_Failcode1
  bus_selector3 : BusSelector  OutputSignals=CAN3_Rr_Failcode2
  bus_selector4 : BusSelector  OutputSignals=CAN3_Rr_Failcodehistory1
  bus_selector5 : BusSelector  OutputSignals=CAN3_Rr_Failcodehistory2
  bus_selector6 : BusSelector  OutputSignals=CAN3_Rr_LLCTemp
  bus_selector7 : BusSelector  OutputSignals=CAN3_Rr_LLCflowReq
  bus_selector8 : BusSelector  OutputSignals=CAN3_Rr_MCUTempWarn
  bus_selector9 : BusSelector  OutputSignals=CAN3_Rr_TMTempWarn
  VHAL_RrCoolanttempReq_cnt : Outport
  VHAL_RrEOPSpdSet_rpm : Outport  Port=2
  VHAL_RrFailcode1_enum : Outport  Port=3
  VHAL_RrFailcode2_enum : Outport  Port=4
  VHAL_RrFailcodehistory1_enum : Outport  Port=5
  VHAL_RrFailcodehistory2_enum : Outport  Port=6
  VHAL_RrLLCTemp_C : Outport  Port=7
  VHAL_RrLLCflowReq_Lpmin : Outport  Port=8
  VHAL_RrMCUTempWarn_enum : Outport  Port=9
  VHAL_RrTMTempWarn_enum : Outport  Port=10
  wires:
  DT_CAN3_SG_MCU_R2/1 -> [DT_CAN3_SG_MCU_R2]
  [DT_CAN3_SG_MCU_R2] -> bus_selector/1
  bus_selector/1 -> RrCoolanttempReq/1(Rr_CoolanttempReq)  "<CAN3_Rr_CoolanttempReq>"
  RrCoolanttempReq/1(VHAL_RrCoolanttempReq_cnt) -> VHAL_RrCoolanttempReq_cnt/1
  [DT_CAN3_SG_MCU_R2] -> bus_selector1/1
  bus_selector1/1 -> RrEOPSpdSet/1(Rr_EOP_SpdSet)  "<CAN3_Rr_EOP_SpdSet>"
  RrEOPSpdSet/1(VHAL_RrEOPSpdSet_rpm) -> VHAL_RrEOPSpdSet_rpm/1
  [DT_CAN3_SG_MCU_R2] -> bus_selector2/1
  bus_selector2/1 -> RrFailcode1/1(Rr_Failcode1)  "<CAN3_Rr_Failcode1>"
  RrFailcode1/1(VHAL_RrFailcode1_enum) -> VHAL_RrFailcode1_enum/1
  [DT_CAN3_SG_MCU_R2] -> bus_selector3/1
  bus_selector3/1 -> RrFailcode2/1(Rr_Failcode2)  "<CAN3_Rr_Failcode2>"
  RrFailcode2/1(VHAL_RrFailcode2_enum) -> VHAL_RrFailcode2_enum/1
  [DT_CAN3_SG_MCU_R2] -> bus_selector4/1
  bus_selector4/1 -> RrFailcodehistory1/1(Rr_Failcodehistory1)  "<CAN3_Rr_Failcodehistory1>"
  RrFailcodehistory1/1(VHAL_RrFailcodehistory1_enum) -> VHAL_RrFailcodehistory1_enum/1
  [DT_CAN3_SG_MCU_R2] -> bus_selector5/1
  bus_selector5/1 -> RrFailcodehistory2/1(Rr_Failcodehistory2)  "<CAN3_Rr_Failcodehistory2>"
  RrFailcodehistory2/1(VHAL_RrFailcodehistory2_enum) -> VHAL_RrFailcodehistory2_enum/1
  [DT_CAN3_SG_MCU_R2] -> bus_selector6/1
  bus_selector6/1 -> RrLLCTemp/1(Rr_LLCTemp)  "<CAN3_Rr_LLCTemp>"
  RrLLCTemp/1(VHAL_RrLLCTemp_C) -> VHAL_RrLLCTemp_C/1
  [DT_CAN3_SG_MCU_R2] -> bus_selector7/1
  bus_selector7/1 -> RrLLCflowReq/1(Rr_LLCflowReq)  "<CAN3_Rr_LLCflowReq>"
  RrLLCflowReq/1(VHAL_RrLLCflowReq_Lpmin) -> VHAL_RrLLCflowReq_Lpmin/1
  [DT_CAN3_SG_MCU_R2] -> bus_selector8/1
  bus_selector8/1 -> RrMCUTempWarn/1(Rr_MCUTempWarn)  "<CAN3_Rr_MCUTempWarn>"
  RrMCUTempWarn/1(VHAL_RrMCUTempWarn_enum) -> VHAL_RrMCUTempWarn_enum/1
  [DT_CAN3_SG_MCU_R2] -> bus_selector9/1
  bus_selector9/1 -> RrTMTempWarn/1(Rr_TMTempWarn)  "<CAN3_Rr_TMTempWarn>"
  RrTMTempWarn/1(VHAL_RrTMTempWarn_enum) -> VHAL_RrTMTempWarn_enum/1

== system halin/HAL_IN/CAN3/Shifter1 ==
  DT_CAN3_SG_Shifter1 : Inport
  0x9d : Constant  Value=0x9d
  0xf9 : Constant  Value=0xf9
  BitwiseAND{,1..3} (4 alike) : simulink/Logic and Bit Operations/Bitwise Operator  logicop=AND  UseBitMask=on  BitMask=0xFF  BitMaskRealWorld=Stored Integer
  BitwiseOR{,1..3} (4 alike) : simulink/Logic and Bit Operations/Bitwise Operator  logicop=OR  UseBitMask=off  BitMask=bin2dec('11011001')  BitMaskRealWorld=Stored Integer
  DDM_CS&RC_Comparison : FVT_lib/hal/DDM_CS&RC_Comparison  MsgCycleTime=100
  Data Type Conversion{,1..3} (4 alike) : DataTypeConversion  OutDataTypeStr=uint8
  KHAL_CAN3Shifter1E2E_flg : Constant  Value=KHAL_CAN3Shifter1E2E_flg
  LeftShift : ArithShift  BitShiftDirection=Left
  LeftShift1 : ArithShift  BitShiftDirection=Left
  LeftShift2 : ArithShift  BitShiftDirection=Left
  LeftShift3 : ArithShift  BitShiftNumber=4  BitShiftDirection=Left
  MessageRollingCounter : FVT_lib/hal/MessageRollingCounter  CounterMAX=14  task_time_ms=5  msg_time_ms=100
  Mux : Mux  Inputs=7
  ShifterCRC8 : Subsystem
  ShifterHandleCmd : Subsystem
  ShifterRC : Subsystem
  bus_selector : BusSelector  OutputSignals=CAN3_Shifter_CRC8,CAN3_Shifter_Fail_sta,CAN3_Shifter_Handle_Cmd,CAN3_Shifter_RC
  bus_selector1 : BusSelector  OutputSignals=CAN3_Shifter_CRC8
  bus_selector2 : BusSelector  OutputSignals=CAN3_Shifter_Handle_Cmd
  bus_selector3 : BusSelector  OutputSignals=CAN3_Shifter_RC
  constant{,1..3} (4 alike) : Constant  Value=0x0  OutDataTypeStr=uint8
  VHAL_Shifter1CSErr_flg : Outport
  VHAL_Shifter1RCErr_flg : Outport  Port=2
  VHAL_ShifterCRC8_enum : Outport  Port=3
  VHAL_ShifterHandleCmd_enum : Outport  Port=4
  VHAL_ShifterRC_enum : Outport  Port=5
  wires:
  DT_CAN3_SG_Shifter1/1 -> [DT_CAN3_SG_Shifter1]
  [DT_CAN3_SG_Shifter1] -> bus_selector/1
  bus_selector/1 -> [CAN3_Shifter_CRC8]  "<CAN3_Shifter_CRC8>"
  [CAN3_Shifter_CRC8] -> LeftShift/1
  LeftShift/1 -> BitwiseAND/1
  BitwiseAND/1 -> [Byte_0_CAN3_Shifter_CRC8]
  bus_selector/2 -> [CAN3_Shifter_Fail_sta]  "<CAN3_Shifter_Fail_sta>"
  [CAN3_Shifter_Fail_sta] -> LeftShift1/1
  LeftShift1/1 -> BitwiseAND1/1
  BitwiseAND1/1 -> [Byte_2_CAN3_Shifter_Fail_sta]
  bus_selector/3 -> [CAN3_Shifter_Handle_Cmd]  "<CAN3_Shifter_Handle_Cmd>"
  [CAN3_Shifter_Handle_Cmd] -> LeftShift2/1
  LeftShift2/1 -> BitwiseAND2/1
  BitwiseAND2/1 -> [Byte_7_CAN3_Shifter_Handle_Cmd]
  bus_selector/4 -> [CAN3_Shifter_RC]  "<CAN3_Shifter_RC>"
  [CAN3_Shifter_RC] -> LeftShift3/1
  LeftShift3/1 -> BitwiseAND3/1
  BitwiseAND3/1 -> [Byte_1_CAN3_Shifter_RC]
  Data Type Conversion/1 -> BitwiseOR/1
  [Byte_0_CAN3_Shifter_CRC8] -> Data Type Conversion/1
  BitwiseOR/1 -> [Byte_0]
  Data Type Conversion1/1 -> BitwiseOR1/1
  [Byte_1_CAN3_Shifter_RC] -> Data Type Conversion1/1
  BitwiseOR1/1 -> [Byte_1]
  Data Type Conversion2/1 -> BitwiseOR2/1
  [Byte_2_CAN3_Shifter_Fail_sta] -> Data Type Conversion2/1
  BitwiseOR2/1 -> [Byte_2]
  constant/1 -> [Byte_3]
  constant1/1 -> [Byte_4]
  constant2/1 -> [Byte_5]
  constant3/1 -> [Byte_6]
  Data Type Conversion3/1 -> BitwiseOR3/1
  [Byte_7_CAN3_Shifter_Handle_Cmd] -> Data Type Conversion3/1
  BitwiseOR3/1 -> [Byte_7]
  [Byte_1] -> Mux/1
  [Byte_2] -> Mux/2
  [Byte_3] -> Mux/3
  [Byte_4] -> Mux/4
  [Byte_5] -> Mux/5
  [Byte_6] -> Mux/6
  [Byte_7] -> Mux/7
  Mux/1 -> [VHAL_CAN3Shifter1noCS_raw]
  KHAL_CAN3Shifter1E2E_flg/1 -> DDM_CS&RC_Comparison/1
  0x9d/1 -> DDM_CS&RC_Comparison/2
  0xf9/1 -> DDM_CS&RC_Comparison/3
  [VHAL_CAN3Shifter1noCS_raw] -> DDM_CS&RC_Comparison/4
  [Byte_0] -> DDM_CS&RC_Comparison/5
  [RC_ECU] -> DDM_CS&RC_Comparison/6
  MessageRollingCounter/1 -> DDM_CS&RC_Comparison/7
  DDM_CS&RC_Comparison/1 -> VHAL_Shifter1CSErr_flg/1
  DDM_CS&RC_Comparison/2 -> VHAL_Shifter1RCErr_flg/1
  [DT_CAN3_SG_Shifter1] -> bus_selector1/1
  bus_selector1/1 -> ShifterCRC8/1(Shifter_CRC8)  "<CAN3_Shifter_CRC8>"
  ShifterCRC8/1(VHAL_ShifterCRC8_enum) -> VHAL_ShifterCRC8_enum/1
  [DT_CAN3_SG_Shifter1] -> bus_selector2/1
  bus_selector2/1 -> ShifterHandleCmd/1(Shifter_Handle_Cmd)  "<CAN3_Shifter_Handle_Cmd>"
  ShifterHandleCmd/1(VHAL_ShifterHandleCmd_enum) -> VHAL_ShifterHandleCmd_enum/1
  [DT_CAN3_SG_Shifter1] -> bus_selector3/1
  bus_selector3/1 -> ShifterRC/1(Shifter_RC)  "<CAN3_Shifter_RC>"
  ShifterRC/1(VHAL_ShifterRC_enum) -> VHAL_ShifterRC_enum/1, [RC_ECU]

== system halin/HAL_IN/CAN3/VHAL_CANMsgInvalidBMS1_flg ==
  Cast To Boolean13 : DataTypeConversion  OutDataTypeStr=boolean
  Constant : Constant  Value=TRUE
  Latch13 : hcu_lib/Basic_Blocks/Latch
  Switch13 : Switch  Criteria=u2 ~= 0
  Unit Delay : UnitDelay  SampleTime=-1  HasFrameUpgradeWarning=on
  UnitConverter : DataTypeConversion  OutDataTypeStr=boolean
  Out : Outport
  wires:
  Constant/1 -> Switch13/3
  Unit Delay/1 -> Cast To Boolean13/1
  Cast To Boolean13/1 -> Switch13/1, Latch13/1
  Switch13/1 -> UnitConverter/1
  Latch13/1 -> Switch13/2
  UnitConverter/1 -> Unit Delay/1, Out/1  "VHAL_CANMsgInvalidBMS1_flg"

== system halin/HAL_IN/CAN3/VHAL_CANMsgInvalidBMS2_flg ==
  Cast To Boolean13 : DataTypeConversion  OutDataTypeStr=boolean
  Constant : Constant  Value=TRUE
  Latch13 : hcu_lib/Basic_Blocks/Latch
  Switch13 : Switch  Criteria=u2 ~= 0
  Unit Delay : UnitDelay  SampleTime=-1  HasFrameUpgradeWarning=on
  UnitConverter : DataTypeConversion  OutDataTypeStr=boolean
  Out : Outport
  wires:
  Constant/1 -> Switch13/3
  Unit Delay/1 -> Cast To Boolean13/1
  Cast To Boolean13/1 -> Switch13/1, Latch13/1
  Switch13/1 -> UnitConverter/1
  Latch13/1 -> Switch13/2
  UnitConverter/1 -> Unit Delay/1, Out/1  "VHAL_CANMsgInvalidBMS2_flg"

== system halin/HAL_IN/CAN3/VHAL_CANMsgInvalidBMS3_flg ==
  Cast To Boolean13 : DataTypeConversion  OutDataTypeStr=boolean
  Constant : Constant  Value=TRUE
  Latch13 : hcu_lib/Basic_Blocks/Latch
  Switch13 : Switch  Criteria=u2 ~= 0
  Unit Delay : UnitDelay  SampleTime=-1  HasFrameUpgradeWarning=on
  UnitConverter : DataTypeConversion  OutDataTypeStr=boolean
  Out : Outport
  wires:
  Constant/1 -> Switch13/3
  Unit Delay/1 -> Cast To Boolean13/1
  Cast To Boolean13/1 -> Switch13/1, Latch13/1
  Switch13/1 -> UnitConverter/1
  Latch13/1 -> Switch13/2
  UnitConverter/1 -> Unit Delay/1, Out/1  "VHAL_CANMsgInvalidBMS3_flg"

== system halin/HAL_IN/CAN3/VHAL_CANMsgInvalidBMS4_flg ==
  Cast To Boolean13 : DataTypeConversion  OutDataTypeStr=boolean
  Constant : Constant  Value=TRUE
  Latch13 : hcu_lib/Basic_Blocks/Latch
  Switch13 : Switch  Criteria=u2 ~= 0
  Unit Delay : UnitDelay  SampleTime=-1  HasFrameUpgradeWarning=on
  UnitConverter : DataTypeConversion  OutDataTypeStr=boolean
  Out : Outport
  wires:
  Constant/1 -> Switch13/3
  Unit Delay/1 -> Cast To Boolean13/1
  Cast To Boolean13/1 -> Switch13/1, Latch13/1
  Switch13/1 -> UnitConverter/1
  Latch13/1 -> Switch13/2
  UnitConverter/1 -> Unit Delay/1, Out/1  "VHAL_CANMsgInvalidBMS4_flg"

== system halin/HAL_IN/CAN3/VHAL_CANMsgInvalidBMS6_flg ==
  Cast To Boolean13 : DataTypeConversion  OutDataTypeStr=boolean
  Constant : Constant  Value=TRUE
  Latch13 : hcu_lib/Basic_Blocks/Latch
  Switch13 : Switch  Criteria=u2 ~= 0
  Unit Delay : UnitDelay  SampleTime=-1  HasFrameUpgradeWarning=on
  UnitConverter : DataTypeConversion  OutDataTypeStr=boolean
  Out : Outport
  wires:
  Constant/1 -> Switch13/3
  Unit Delay/1 -> Cast To Boolean13/1
  Cast To Boolean13/1 -> Switch13/1, Latch13/1
  Switch13/1 -> UnitConverter/1
  Latch13/1 -> Switch13/2
  UnitConverter/1 -> Unit Delay/1, Out/1  "VHAL_CANMsgInvalidBMS6_flg"

== system halin/HAL_IN/CAN3/VHAL_CANMsgInvalidBMS7_flg ==
  Cast To Boolean13 : DataTypeConversion  OutDataTypeStr=boolean
  Constant : Constant  Value=TRUE
  Latch13 : hcu_lib/Basic_Blocks/Latch
  Switch13 : Switch  Criteria=u2 ~= 0
  Unit Delay : UnitDelay  SampleTime=-1  HasFrameUpgradeWarning=on
  UnitConverter : DataTypeConversion  OutDataTypeStr=boolean
  Out : Outport
  wires:
  Constant/1 -> Switch13/3
  Unit Delay/1 -> Cast To Boolean13/1
  Cast To Boolean13/1 -> Switch13/1, Latch13/1
  Switch13/1 -> UnitConverter/1
  Latch13/1 -> Switch13/2
  UnitConverter/1 -> Unit Delay/1, Out/1  "VHAL_CANMsgInvalidBMS7_flg"

== system halin/HAL_IN/CAN3/VHAL_CANMsgInvalidCCU1_flg ==
  Cast To Boolean13 : DataTypeConversion  OutDataTypeStr=boolean
  Constant : Constant  Value=TRUE
  Latch13 : hcu_lib/Basic_Blocks/Latch
  Switch13 : Switch  Criteria=u2 ~= 0
  Unit Delay : UnitDelay  SampleTime=-1  HasFrameUpgradeWarning=on
  UnitConverter : DataTypeConversion  OutDataTypeStr=boolean
  Out : Outport
  wires:
  Constant/1 -> Switch13/3
  Unit Delay/1 -> Cast To Boolean13/1
  Cast To Boolean13/1 -> Switch13/1, Latch13/1
  Switch13/1 -> UnitConverter/1
  Latch13/1 -> Switch13/2
  UnitConverter/1 -> Unit Delay/1, Out/1  "VHAL_CANMsgInvalidCCU1_flg"

== system halin/HAL_IN/CAN3/VHAL_CANMsgInvalidCCU2_flg ==
  Cast To Boolean13 : DataTypeConversion  OutDataTypeStr=boolean
  Constant : Constant  Value=TRUE
  Latch13 : hcu_lib/Basic_Blocks/Latch
  Switch13 : Switch  Criteria=u2 ~= 0
  Unit Delay : UnitDelay  SampleTime=-1  HasFrameUpgradeWarning=on
  UnitConverter : DataTypeConversion  OutDataTypeStr=boolean
  Out : Outport
  wires:
  Constant/1 -> Switch13/3
  Unit Delay/1 -> Cast To Boolean13/1
  Cast To Boolean13/1 -> Switch13/1, Latch13/1
  Switch13/1 -> UnitConverter/1
  Latch13/1 -> Switch13/2
  UnitConverter/1 -> Unit Delay/1, Out/1  "VHAL_CANMsgInvalidCCU2_flg"

== system halin/HAL_IN/CAN3/VHAL_CANMsgInvalidCCU4_flg ==
  Cast To Boolean13 : DataTypeConversion  OutDataTypeStr=boolean
  Constant : Constant  Value=TRUE
  Latch13 : hcu_lib/Basic_Blocks/Latch
  Switch13 : Switch  Criteria=u2 ~= 0
  Unit Delay : UnitDelay  SampleTime=-1  HasFrameUpgradeWarning=on
  UnitConverter : DataTypeConversion  OutDataTypeStr=boolean
  Out : Outport
  wires:
  Constant/1 -> Switch13/3
  Unit Delay/1 -> Cast To Boolean13/1
  Cast To Boolean13/1 -> Switch13/1, Latch13/1
  Switch13/1 -> UnitConverter/1
  Latch13/1 -> Switch13/2
  UnitConverter/1 -> Unit Delay/1, Out/1  "VHAL_CANMsgInvalidCCU4_flg"

== system halin/HAL_IN/CAN3/VHAL_CANMsgInvalidMCUF1_flg ==
  Cast To Boolean13 : DataTypeConversion  OutDataTypeStr=boolean
  Constant : Constant  Value=TRUE
  Latch13 : hcu_lib/Basic_Blocks/Latch
  Switch13 : Switch  Criteria=u2 ~= 0
  Unit Delay : UnitDelay  SampleTime=-1  HasFrameUpgradeWarning=on
  UnitConverter : DataTypeConversion  OutDataTypeStr=boolean
  Out : Outport
  wires:
  Constant/1 -> Switch13/3
  Unit Delay/1 -> Cast To Boolean13/1
  Cast To Boolean13/1 -> Switch13/1, Latch13/1
  Switch13/1 -> UnitConverter/1
  Latch13/1 -> Switch13/2
  UnitConverter/1 -> Unit Delay/1, Out/1  "VHAL_CANMsgInvalidMCUF1_flg"

== system halin/HAL_IN/CAN3/VHAL_CANMsgInvalidMCUF2_flg ==
  Cast To Boolean13 : DataTypeConversion  OutDataTypeStr=boolean
  Constant : Constant  Value=TRUE
  Latch13 : hcu_lib/Basic_Blocks/Latch
  Switch13 : Switch  Criteria=u2 ~= 0
  Unit Delay : UnitDelay  SampleTime=-1  HasFrameUpgradeWarning=on
  UnitConverter : DataTypeConversion  OutDataTypeStr=boolean
  Out : Outport
  wires:
  Constant/1 -> Switch13/3
  Unit Delay/1 -> Cast To Boolean13/1
  Cast To Boolean13/1 -> Switch13/1, Latch13/1
  Switch13/1 -> UnitConverter/1
  Latch13/1 -> Switch13/2
  UnitConverter/1 -> Unit Delay/1, Out/1  "VHAL_CANMsgInvalidMCUF2_flg"

== system halin/HAL_IN/CAN3/VHAL_CANMsgInvalidMCUR1_flg ==
  Cast To Boolean13 : DataTypeConversion  OutDataTypeStr=boolean
  Constant : Constant  Value=TRUE
  Latch13 : hcu_lib/Basic_Blocks/Latch
  Switch13 : Switch  Criteria=u2 ~= 0
  Unit Delay : UnitDelay  SampleTime=-1  HasFrameUpgradeWarning=on
  UnitConverter : DataTypeConversion  OutDataTypeStr=boolean
  Out : Outport
  wires:
  Constant/1 -> Switch13/3
  Unit Delay/1 -> Cast To Boolean13/1
  Cast To Boolean13/1 -> Switch13/1, Latch13/1
  Switch13/1 -> UnitConverter/1
  Latch13/1 -> Switch13/2
  UnitConverter/1 -> Unit Delay/1, Out/1  "VHAL_CANMsgInvalidMCUR1_flg"

== system halin/HAL_IN/CAN3/VHAL_CANMsgInvalidMCUR2_flg ==
  Cast To Boolean13 : DataTypeConversion  OutDataTypeStr=boolean
  Constant : Constant  Value=TRUE
  Latch13 : hcu_lib/Basic_Blocks/Latch
  Switch13 : Switch  Criteria=u2 ~= 0
  Unit Delay : UnitDelay  SampleTime=-1  HasFrameUpgradeWarning=on
  UnitConverter : DataTypeConversion  OutDataTypeStr=boolean
  Out : Outport
  wires:
  Constant/1 -> Switch13/3
  Unit Delay/1 -> Cast To Boolean13/1
  Cast To Boolean13/1 -> Switch13/1, Latch13/1
  Switch13/1 -> UnitConverter/1
  Latch13/1 -> Switch13/2
  UnitConverter/1 -> Unit Delay/1, Out/1  "VHAL_CANMsgInvalidMCUR2_flg"

== system halin/HAL_IN/CAN3/VHAL_CANMsgInvalidShifter1_flg ==
  Cast To Boolean13 : DataTypeConversion  OutDataTypeStr=boolean
  Constant : Constant  Value=TRUE
  Latch13 : hcu_lib/Basic_Blocks/Latch
  Switch13 : Switch  Criteria=u2 ~= 0
  Unit Delay : UnitDelay  SampleTime=-1  HasFrameUpgradeWarning=on
  UnitConverter : DataTypeConversion  OutDataTypeStr=boolean
  Out : Outport
  wires:
  Constant/1 -> Switch13/3
  Unit Delay/1 -> Cast To Boolean13/1
  Cast To Boolean13/1 -> Switch13/1, Latch13/1
  Switch13/1 -> UnitConverter/1
  Latch13/1 -> Switch13/2
  UnitConverter/1 -> Unit Delay/1, Out/1  "VHAL_CANMsgInvalidShifter1_flg"

== system halin/HAL_IN/CAN4/DKC1 ==
  DT_CAN4_SG_DKC1 : Inport
  DKCReVehData : Subsystem
  DKCRemotePW : Subsystem
  PCommandToBCM : Subsystem
  PCommandToPTG : Subsystem
  PDKeyAreaLockUnlock : Subsystem
  PDKeyAreaPS : Subsystem
  PDKeyAreaPTG : Subsystem
  PDKeyWelcome : Subsystem
  PDkeyShowIVI : Subsystem
  PKeyMiss : Subsystem
  PKeyMode : Subsystem
  PUIDLowPower : Subsystem
  bus_selector : BusSelector  OutputSignals=CAN4_DKC_Re_VehData
  bus_selector1 : BusSelector  OutputSignals=CAN4_DKC_Remote_PW
  bus_selector10 : BusSelector  OutputSignals=CAN4_P_KeyMode
  bus_selector11 : BusSelector  OutputSignals=CAN4_P_UID_LowPower
  bus_selector2 : BusSelector  OutputSignals=CAN4_P_CommandToBCM
  bus_selector3 : BusSelector  OutputSignals=CAN4_P_CommandToPTG
  bus_selector4 : BusSelector  OutputSignals=CAN4_P_DKey_Area_LockUnlock
  bus_selector5 : BusSelector  OutputSignals=CAN4_P_DKey_Area_PS
  bus_selector6 : BusSelector  OutputSignals=CAN4_P_DKey_Area_PTG
  bus_selector7 : BusSelector  OutputSignals=CAN4_P_DKey_Welcome
  bus_selector8 : BusSelector  OutputSignals=CAN4_P_Dkey_Show_IVI
  bus_selector9 : BusSelector  OutputSignals=CAN4_P_KeyMiss
  VHAL_DKCReVehData_enum : Outport
  VHAL_DKCRemotePW_enum : Outport  Port=2
  VHAL_PCommandToBCM_enum : Outport  Port=3
  VHAL_PCommandToPTG_enum : Outport  Port=4
  VHAL_PDKeyAreaLockUnlock_enum : Outport  Port=5
  VHAL_PDKeyAreaPS_enum : Outport  Port=6
  VHAL_PDKeyAreaPTG_enum : Outport  Port=7
  VHAL_PDKeyWelcome_enum : Outport  Port=8
  VHAL_PDkeyShowIVI_enum : Outport  Port=9
  VHAL_PKeyMiss_flg : Outport  Port=10
  VHAL_PKeyMode_enum : Outport  Port=11
  VHAL_PUIDLowPower_flg : Outport  Port=12
  wires:
  DT_CAN4_SG_DKC1/1 -> [DT_CAN4_SG_DKC1]
  [DT_CAN4_SG_DKC1] -> bus_selector/1
  bus_selector/1 -> DKCReVehData/1(DKC_Re_VehData)  "<CAN4_DKC_Re_VehData>"
  DKCReVehData/1(VHAL_DKCReVehData_enum) -> VHAL_DKCReVehData_enum/1
  [DT_CAN4_SG_DKC1] -> bus_selector1/1
  bus_selector1/1 -> DKCRemotePW/1(DKC_Remote_PW)  "<CAN4_DKC_Remote_PW>"
  DKCRemotePW/1(VHAL_DKCRemotePW_enum) -> VHAL_DKCRemotePW_enum/1
  [DT_CAN4_SG_DKC1] -> bus_selector2/1
  bus_selector2/1 -> PCommandToBCM/1(P_CommandToBCM)  "<CAN4_P_CommandToBCM>"
  PCommandToBCM/1(VHAL_PCommandToBCM_enum) -> VHAL_PCommandToBCM_enum/1
  [DT_CAN4_SG_DKC1] -> bus_selector3/1
  bus_selector3/1 -> PCommandToPTG/1(P_CommandToPTG)  "<CAN4_P_CommandToPTG>"
  PCommandToPTG/1(VHAL_PCommandToPTG_enum) -> VHAL_PCommandToPTG_enum/1
  [DT_CAN4_SG_DKC1] -> bus_selector4/1
  bus_selector4/1 -> PDKeyAreaLockUnlock/1(P_DKey_Area_LockUnlock)  "<CAN4_P_DKey_Area_LockUnlock>"
  PDKeyAreaLockUnlock/1(VHAL_PDKeyAreaLockUnlock_enum) -> VHAL_PDKeyAreaLockUnlock_enum/1
  [DT_CAN4_SG_DKC1] -> bus_selector5/1
  bus_selector5/1 -> PDKeyAreaPS/1(P_DKey_Area_PS)  "<CAN4_P_DKey_Area_PS>"
  PDKeyAreaPS/1(VHAL_PDKeyAreaPS_enum) -> VHAL_PDKeyAreaPS_enum/1
  [DT_CAN4_SG_DKC1] -> bus_selector6/1
  bus_selector6/1 -> PDKeyAreaPTG/1(P_DKey_Area_PTG)  "<CAN4_P_DKey_Area_PTG>"
  PDKeyAreaPTG/1(VHAL_PDKeyAreaPTG_enum) -> VHAL_PDKeyAreaPTG_enum/1
  [DT_CAN4_SG_DKC1] -> bus_selector7/1
  bus_selector7/1 -> PDKeyWelcome/1(P_DKey_Welcome)  "<CAN4_P_DKey_Welcome>"
  PDKeyWelcome/1(VHAL_PDKeyWelcome_enum) -> VHAL_PDKeyWelcome_enum/1
  [DT_CAN4_SG_DKC1] -> bus_selector8/1
  bus_selector8/1 -> PDkeyShowIVI/1(P_Dkey_Show_IVI)  "<CAN4_P_Dkey_Show_IVI>"
  PDkeyShowIVI/1(VHAL_PDkeyShowIVI_enum) -> VHAL_PDkeyShowIVI_enum/1
  [DT_CAN4_SG_DKC1] -> bus_selector9/1
  bus_selector9/1 -> PKeyMiss/1(P_KeyMiss)  "<CAN4_P_KeyMiss>"
  PKeyMiss/1(VHAL_PKeyMiss_flg) -> VHAL_PKeyMiss_flg/1
  [DT_CAN4_SG_DKC1] -> bus_selector10/1
  bus_selector10/1 -> PKeyMode/1(P_KeyMode)  "<CAN4_P_KeyMode>"
  PKeyMode/1(VHAL_PKeyMode_enum) -> VHAL_PKeyMode_enum/1
  [DT_CAN4_SG_DKC1] -> bus_selector11/1
  bus_selector11/1 -> PUIDLowPower/1(P_UID_LowPower)  "<CAN4_P_UID_LowPower>"
  PUIDLowPower/1(VHAL_PUIDLowPower_flg) -> VHAL_PUIDLowPower_flg/1

== system halin/HAL_IN/CAN4/DKC2 ==
  DT_CAN4_SG_DKC2 : Inport
  EncryptionDATA063 : Subsystem
  EncryptionDATA64127 : Subsystem
  RandomNumberX : Subsystem
  bus_selector : BusSelector  OutputSignals=CAN4_EncryptionDATA_0_63
  bus_selector1 : BusSelector  OutputSignals=CAN4_EncryptionDATA_64_127
  bus_selector2 : BusSelector  OutputSignals=CAN4_Random_Number_X
  VHAL_EncryptionDATA063_enum : Outport
  VHAL_EncryptionDATA64127_enum : Outport  Port=2
  VHAL_RandomNumberX_enum : Outport  Port=3
  wires:
  DT_CAN4_SG_DKC2/1 -> [DT_CAN4_SG_DKC2]
  [DT_CAN4_SG_DKC2] -> bus_selector/1
  bus_selector/1 -> EncryptionDATA063/1(EncryptionDATA_0_63)  "<CAN4_EncryptionDATA_0_63>"
  EncryptionDATA063/1(VHAL_EncryptionDATA063_enum) -> VHAL_EncryptionDATA063_enum/1
  [DT_CAN4_SG_DKC2] -> bus_selector1/1
  bus_selector1/1 -> EncryptionDATA64127/1(EncryptionDATA_64_127)  "<CAN4_EncryptionDATA_64_127>"
  EncryptionDATA64127/1(VHAL_EncryptionDATA64127_enum) -> VHAL_EncryptionDATA64127_enum/1
  [DT_CAN4_SG_DKC2] -> bus_selector2/1
  bus_selector2/1 -> RandomNumberX/1(Random_Number_X)  "<CAN4_Random_Number_X>"
  RandomNumberX/1(VHAL_RandomNumberX_enum) -> VHAL_RandomNumberX_enum/1

== system halin/HAL_IN/CAN4/GW_ZDR_PTG1 ==
  DT_CAN4_SG_GW_ZDR_PTG1 : Inport
  PTGRDILSta : Subsystem
  bus_selector : BusSelector  OutputSignals=CAN4_PTG_RDIL_Sta
  VHAL_PTGRDILSta_enum : Outport
  wires:
  DT_CAN4_SG_GW_ZDR_PTG1/1 -> [DT_CAN4_SG_GW_ZDR_PTG1]
  [DT_CAN4_SG_GW_ZDR_PTG1] -> bus_selector/1
  bus_selector/1 -> PTGRDILSta/1(PTG_RDIL_Sta)  "<CAN4_PTG_RDIL_Sta>"
  PTGRDILSta/1(VHAL_PTGRDILSta_enum) -> VHAL_PTGRDILSta_enum/1
